simulink model "thermostatslx"  (R2019a)
settings: Solver=ode45  StartTime=0.0  StopTime=20  MaxStep=0.0001  RelTol=1e-5  AbsTol=1e-8
undefined symbols (not defined in the file or in its folder): normrnd
Description:
  | Bouncing Ball Model
  | 
  | This model calculates the trajectory, over time, of a ball thrown
  | upward with a velocity of 15 meters per second from a height of 10 m.
  | The position of the ball is plotted in the upper axis of the scope while
  | the velocity of the ball is plotted in the lower axis. For the
  | recommended approach to modeling a bouncing ball, type
  | 'sldemo_bounce' at the MATLAB prompt.
settings Model: ExtModeTrigMode=oneshot  ExtModeArmWhenConnect=off  ExtModeAutoUpdateStatusClock=off  Creator=The MathWorks, Inc.  LastModifiedBy=Mojzar
settings SolverCC: AutoScaleAbsTol=off  ZeroCrossAlgorithm=Adaptive
settings DataIOCC: ExternalInput=[]  InitialState=[]  MaxDataPoints=7500  SaveFormat=Array  SaveOutput=off  SignalLogging=off  DSMLogging=off  SaveTime=off
settings OptimizationCC: BooleanDataType=off  ExpressionDepthLimit=2147483647  InitFltsAndDblsToZero=on  LifeSpan=inf  BufferReusableBoundary=off
settings DebuggingCC: SaveWithParameterizedLinksMsg=none  UnderspecifiedInitializationDetection=Classic  MergeDetectMultiDrivingBlocksExec=none  SignalResolutionControl=TryResolveAllWithWarning  IgnoredZcDiagnostic=none  InheritedTsInSrcMsg=none  MultiTaskDSMMsg=warning  MultiTaskCondExecSysMsg=none  SigSpecEnsureSampleTimeMsg=none  FcnCallInpInsideContextMsg=warning  BusObjectLabelMismatch=none  StateNameClashWarn=warning  SFUnexpectedBacktrackingDiag=warning  SFNoUnconditionalDefaultTransitionDiag=warning  SFExecutionAtInitializationDiag=none  ArithmeticOperatorsInVariantConditions=warning
settings HardwareCC: ProdBitPerPointer=32  ProdBitPerSizeT=32  ProdBitPerPtrDiffT=32  ProdLargestAtomicFloat=None  ProdIntDivRoundTo=Undefined  ProdEndianess=Unspecified  ProdWordSize=32  ProdHWDeviceType=32-bit Generic  TargetBitPerPointer=64  TargetBitPerSizeT=64  TargetBitPerPtrDiffT=64  TargetLongLongMode=on  TargetIntDivRoundTo=Zero  TargetEndianess=LittleEndian  TargetWordSize=64  TargetHWDeviceType=MATLAB Host  ProdEqTarget=off
settings ModelReferenceCC: PropagateSignalLabelsOutOfModel=off
settings SFSimCC: SimUseLocalCustomCode=off
settings RTWCC: SystemTargetFile=rsim.tlc  TemplateMakefile=rsim_default_tmf  Description=Rapid Simulation Target  RTWUseLocalCustomCode=off
settings CodeAppCC: StateflowObjectComments=on
settings RSimTargetCC: PreserveStateflowLocalDataDimensions=off
settings ConfigComp: CovMetricSettings=d  CovHtmlReporting=on  CovSaveCumulativeToWorkspaceVar=on  CovSaveSingleToWorkspaceVar=on  CovExternalEMLEnable=off

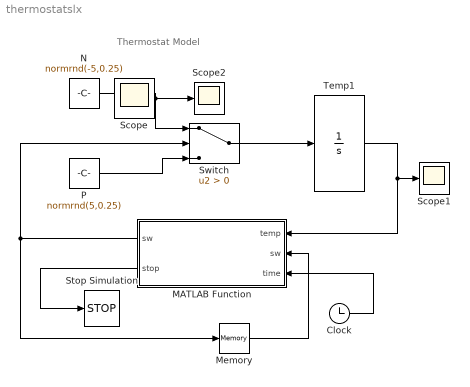
== system thermostatslx ==
  note: Thermostat Model
  Clock : Clock
  MATLAB Function : MATLAB Function  TreatAsAtomicUnit=on
  Memory : Memory  InitialCondition=1
  N : Constant  Value=normrnd(-5,0.25)
  P : Constant  Value=normrnd(5,0.25)
  Scope1 : Scope
  Scope2 : Scope
  Stop Simulation : Stop
  Switch : Switch  Criteria=u2 > Threshold
  Temp1 : Integrator  InitialCondition=25  ZeroCross=off
  Scope : Scope
  wires:
  Switch/1 -> Temp1/1
  P/1 -> Switch/3
  N/1 -> Scope2/1, Switch/1
  Memory/1 -> MATLAB Function/2("sw ")
  MATLAB Function/1(sw) -> Memory/1, Switch/2
  MATLAB Function/2(stop) -> Stop Simulation/1
  Temp1/1 -> Scope1/1, MATLAB Function/1(temp)
  Clock/1 -> MATLAB Function/3(time)

== matlab function thermostatslx/MATLAB Function ==
  data: temp input; sw input; sw output; stop output; time input
function [sw,stop] = fcn(temp,sw,time)
if sw ==1 && temp < 15
    sw = sw - 1;
elseif sw == 0 && temp > 40
    sw = sw +1;
end
stop = 0;
if temp < 25 && time > 8
    stop = 1;
end
